simulink model "ballAndBeam_project_simulations"  (R2020b)
settings: Solver=VariableStepAuto  StartTime=0.0  StopTime=20  RelTol=1e-3
values from neighbouring files (symbols this model uses):
  A = [0,     0,      1,    0 ... (first row only)    [ballAndBeam_project.m]
  Aobs = A - L*C    [ballAndBeam_project.m]
  Aocc = [A-L*C-B*K4+L*D*K4 -B*Kpre4+L*D*Kpre4; zeros(1,n) 0]    [ballAndBeam_project.m]
  B = [0 ... (first row only)    [ballAndBeam_project.m]
  Bobs = [B-L*D L]    [ballAndBeam_project.m]
  Bocc = [zeros(n,1) L; 1 -1]    [ballAndBeam_project.m]
  C = [0 1 0 0]    [ballAndBeam_project.m]
  Cobs = eye(n)    [ballAndBeam_project.m]
  Cocc = [-K4 -Kpre4]    [ballAndBeam_project.m]
  D = 0    [ballAndBeam_project.m]
  Dobs = zeros(n,2)    [ballAndBeam_project.m]
  Docc = zeros(1,2)    [ballAndBeam_project.m]
  IP = 0.8    [ballAndBeam_project.m]
  K1 = place(A,B,Polescl)    [ballAndBeam_project.m]
  K2 = place(A,B,Polescl)    [ballAndBeam_project.m]
  K4 = Kext(1:n)    [ballAndBeam_project.m]
  Kpre1 = inv(-(C-D*K1)*inv(A-B*K1)*B + D)    [ballAndBeam_project.m]
  Kpre2 = inv(-(C-D*K2)*inv(A-B*K2)*B + D)    [ballAndBeam_project.m]
  Kpre3 = inv(-(C-D*K3)*inv(A-B*K3)*B + D)    [ballAndBeam_project.m]
  Kpre4 = Kext(n+1)    [ballAndBeam_project.m]
  n = size(A,1)    [ballAndBeam_project.m]
  OP = 0.1    [ballAndBeam_project.m]
  S = 1.1    [ballAndBeam_project.m]
undefined symbols (not defined in the file or in its folder): K3
settings Model: Creator=chris  LastModifiedBy=chris

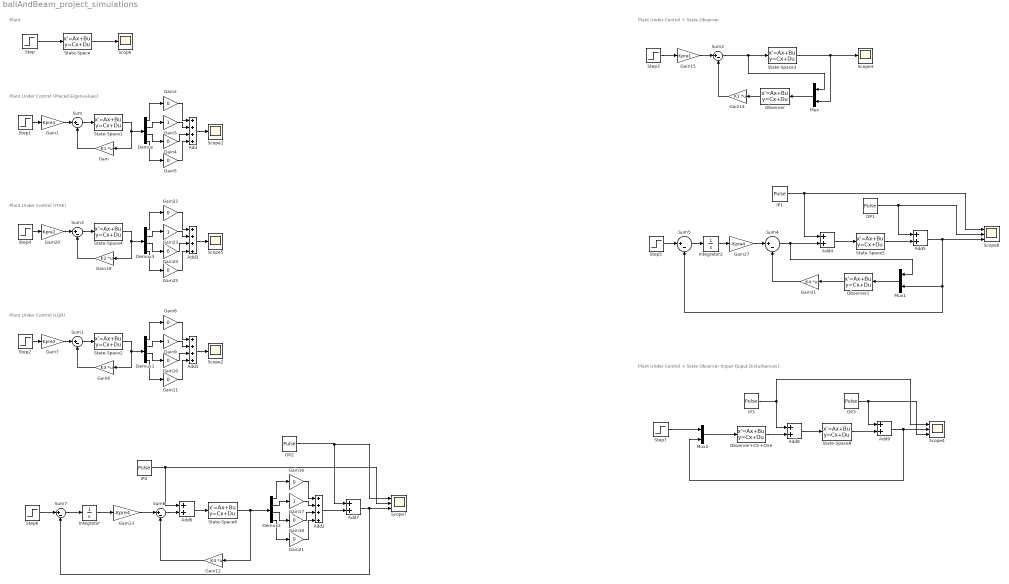
== system ballAndBeam_project_simulations ==
  note: Plant Under Control + State Observer
  note: Plant
  note: Plant Under Control (Placed Eigenvalues)
  note: Plant Under Control (LQR)
  note: Plant Under Control (ITAE)
  note: Plant Under Control + State Observer (Input-Ouput Disturbances)
  Add{,1..3} (4 alike) : Sum  Inputs=++++
  Add{4..9} (6 alike) : Sum
  Demux{,1..3} (4 alike) : Demux
  Gain : Gain  Gain=K1  Multiplication=Matrix(K*u)
  Gain1 : Gain  Gain=Kpre1
  Gain{2,4..5,8,10..11,16,18,21..22,24..25} (12 alike) : Gain  Gain=0
  Gain12 : Gain  Gain=K4  Multiplication=Matrix(K*u)
  Gain13 : Gain  Gain=-Kpre4
  Gain14 : Gain  Gain=K1  Multiplication=Matrix(K*u)
  Gain15 : Gain  Gain=Kpre1
  Gain{3,9,17,23} (4 alike) : Gain
  Gain19 : Gain  Gain=K2  Multiplication=Matrix(K*u)
  Gain20 : Gain  Gain=Kpre2
  Gain27 : Gain  Gain=-Kpre4
  Gain31 : Gain  Gain=K4  Multiplication=Matrix(K*u)
  Gain6 : Gain  Gain=K3  Multiplication=Matrix(K*u)
  Gain7 : Gain  Gain=Kpre3
  IP1 : DiscretePulseGenerator  PulseType=Time based  Amplitude=IP  Period=20  PulseWidth=15  PhaseDelay=12
  IP2 : DiscretePulseGenerator  PulseType=Time based  Amplitude=IP  Period=20  PulseWidth=15  PhaseDelay=12
  IP3 : DiscretePulseGenerator  PulseType=Time based  Amplitude=IP  Period=20  PulseWidth=15  PhaseDelay=12
  Integrator : Integrator
  Integrator2 : Integrator
  Mux : Mux  Inputs=2
  Mux1 : Mux  Inputs=2
  Mux2 : Mux  Inputs=2
  OP1 : DiscretePulseGenerator  PulseType=Time based  Amplitude=OP  Period=20  PulseWidth=10  PhaseDelay=5
  OP2 : DiscretePulseGenerator  PulseType=Time based  Amplitude=OP  Period=20  PulseWidth=10  PhaseDelay=5
  OP3 : DiscretePulseGenerator  PulseType=Time based  Amplitude=OP  Period=20  PulseWidth=10  PhaseDelay=5
  Observer : StateSpace  A=Aobs  B=Bobs  C=Cobs  D=Dobs  InitialCondition=0
  Observer+Ctr+Ctre : StateSpace  A=Aocc  B=Bocc  C=Cocc  D=Docc  InitialCondition=0
  Observer1 : StateSpace  A=Aobs  B=Bobs  C=Cobs  D=Dobs  InitialCondition=0
  Scope{,1..3,5} (5 alike) : Scope
  Scope4 : Scope  NumInputPorts=3
  Scope6 : Scope  NumInputPorts=3
  Scope7 : Scope  NumInputPorts=3
  State-Space : StateSpace  A=A  B=B  C=C  D=D  InitialCondition=0
  State-Space1 : StateSpace  A=A  B=B  C=eye(n)  D=zeros(n,1)  InitialCondition=0
  State-Space2 : StateSpace  A=A  B=B  C=eye(n)  D=zeros(n,1)  InitialCondition=0
  State-Space3 : StateSpace  A=A  B=B  C=C  D=D  InitialCondition=0
  State-Space4 : StateSpace  A=A  B=B  C=eye(n)  D=zeros(n,1)  InitialCondition=0
  State-Space5 : StateSpace  A=1.1*A  B=1.1*B  C=1.1*C  D=1.1*D  InitialCondition=0
  State-Space6 : StateSpace  A=S*A  B=S*B  C=S*eye(n)  D=S*zeros(n,1)  InitialCondition=0
  State-Space8 : StateSpace  A=A  B=B  C=C  D=D  InitialCondition=0
  Step{,1..4,6} (6 alike) : Step  Time=0  SampleTime=0
  Step5 : Step  SampleTime=0
  Step7 : Step  SampleTime=0
  Sum{,1..7} (8 alike) : Sum  Inputs=|+-
  wires:
  Step/1 -> State-Space/1
  State-Space/1 -> Scope/1
  State-Space1/1 -> Gain/1, Demux/1
  Sum/1 -> State-Space1/1
  Gain/1 -> Sum/2
  Step1/1 -> Gain1/1
  Gain1/1 -> Sum/1
  Demux/2 -> Gain3/1
  Demux/1 -> Gain2/1
  Demux/3 -> Gain4/1
  Gain3/1 -> Add/2
  Add/1 -> Scope1/1
  Gain4/1 -> Add/3
  Gain2/1 -> Add/1
  Demux/4 -> Gain5/1
  Gain5/1 -> Add/4
  Add1/1 -> Scope2/1
  Gain9/1 -> Add1/2
  Gain10/1 -> Add1/3
  Gain6/1 -> Sum1/2
  State-Space2/1 -> Gain6/1, Demux1/1
  Demux1/4 -> Gain11/1
  Gain11/1 -> Add1/4
  Gain7/1 -> Sum1/1
  Demux1/1 -> Gain8/1
  Demux1/3 -> Gain10/1
  Sum1/1 -> State-Space2/1
  Demux1/2 -> Gain9/1
  Gain8/1 -> Add1/1
  Step2/1 -> Gain7/1
  Sum2/1 -> Mux/1, State-Space3/1
  Step3/1 -> Gain15/1
  Gain15/1 -> Sum2/1
  State-Space3/1 -> Scope3/1, Mux/2
  Mux/1 -> Observer/1
  Observer/1 -> Gain14/1
  Gain14/1 -> Sum2/2
  Add3/1 -> Scope5/1
  Gain23/1 -> Add3/2
  Gain24/1 -> Add3/3
  Gain19/1 -> Sum3/2
  State-Space4/1 -> Gain19/1, Demux3/1
  Demux3/4 -> Gain25/1
  Gain25/1 -> Add3/4
  Gain20/1 -> Sum3/1
  Demux3/1 -> Gain22/1
  Demux3/3 -> Gain24/1
  Sum3/1 -> State-Space4/1
  Demux3/2 -> Gain23/1
  Gain22/1 -> Add3/1
  Step4/1 -> Gain20/1
  Gain31/1 -> Sum4/2
  Integrator2/1 -> Gain27/1
  Add5/1 -> Scope6/3, Mux1/2, Sum5/2
  Sum5/1 -> Integrator2/1
  Step5/1 -> Sum5/1
  Add4/1 -> State-Space5/1
  Gain27/1 -> Sum4/1
  Observer1/1 -> Gain31/1
  Mux1/1 -> Observer1/1
  Sum4/1 -> Mux1/1, Add4/2
  IP1/1 -> Scope6/1, Add4/1
  State-Space5/1 -> Add5/2
  OP1/1 -> Scope6/2, Add5/1
  Gain17/1 -> Add2/2
  Gain18/1 -> Add2/3
  Gain12/1 -> Sum6/2
  Demux2/4 -> Gain21/1
  Gain21/1 -> Add2/4
  Gain13/1 -> Sum6/1
  Demux2/1 -> Gain16/1
  Demux2/3 -> Gain18/1
  Demux2/2 -> Gain17/1
  Gain16/1 -> Add2/1
  Step6/1 -> Sum7/1
  Sum7/1 -> Integrator/1
  Integrator/1 -> Gain13/1
  Sum6/1 -> Add6/2
  Add6/1 -> State-Space6/1
  State-Space6/1 -> Gain12/1, Demux2/1
  Add2/1 -> Add7/2
  Add7/1 -> Scope7/3, Sum7/2
  IP2/1 -> Scope7/2, Add6/1
  OP2/1 -> Scope7/1, Add7/1
  Step7/1 -> Mux2/1
  Mux2/1 -> Observer+Ctr+Ctre/1
  Observer+Ctr+Ctre/1 -> Add8/2
  Add8/1 -> State-Space8/1
  State-Space8/1 -> Add9/2
  Add9/1 -> Scope4/2, Mux2/2
  IP3/1 -> Scope4/1, Add8/1
  OP3/1 -> Add9/1, Scope4/3
